simulink model "BACKSTEPPINGmasModosDeslisantes"  (R2025a)
settings: Solver=VariableStepAuto  StartTime=0.0  StopTime=10.0  RelTol=1e-3
InitFcn:
  | % --- INICIO DEL CÓDIGO InitFcn ---
  | 
  | % 1. (¡CAMBIA ESTO!) Asegúrate de que esta ruta sea correcta
  | addpath('C:/RoboDK/Matlab/');
  | 
  | % 2. Declarar las variables como globales para que Simulink las vea
  | global RDK;
  | global ROBOT;
  | 
  | % 3. Iniciar la conexión con RoboDK
  | RDK = Robolink();
  | 
  | % 4. (¡CAMBIA ESTO!) Pon el nombre exacto de tu robot en RoboDK
  | robot_name = 'Fanuc CRX-5iA';
  | ROBOT = RDK.Item(robot_name, RDK.ITEM_TYPE_ROBOT);
  | 
  | % 5. Comprobar que se encontró
  | if ~ROBOT.Valid()
  |     % Si el script falla aquí, es porque no encontró tu robot.
  |     error('No se encontró el robot: %s', robot_name);
  | end
  | 
  | % 6. Configurar el modo para simulación en tiempo real
  | RDK.setRunMode(RDK.RUNMODE_SIMULATE);
  | 
  | % 7. Mensaje de éxito
  | fprintf('¡RoboDK y el robot "%s" conectados a Simulink!\n', robot_name);
  | 
  | % --- FIN DEL CÓDIGO ---
libraries: robotmaniplib x1, robotsim3dlib x1, sim3dlib x1
settings Model: Creator=Sandro  LastModifiedBy=jaros

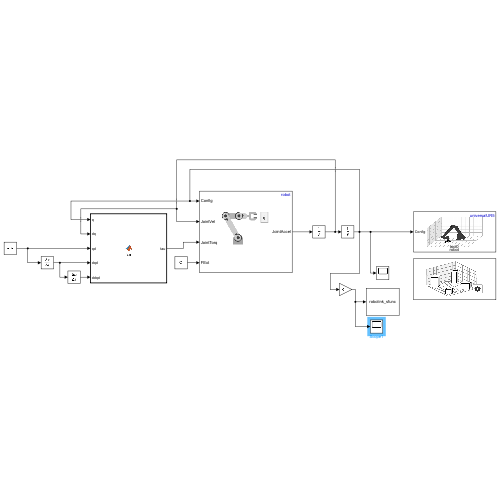
[thumbnail: Simulink's stored preview of the top-level diagram]
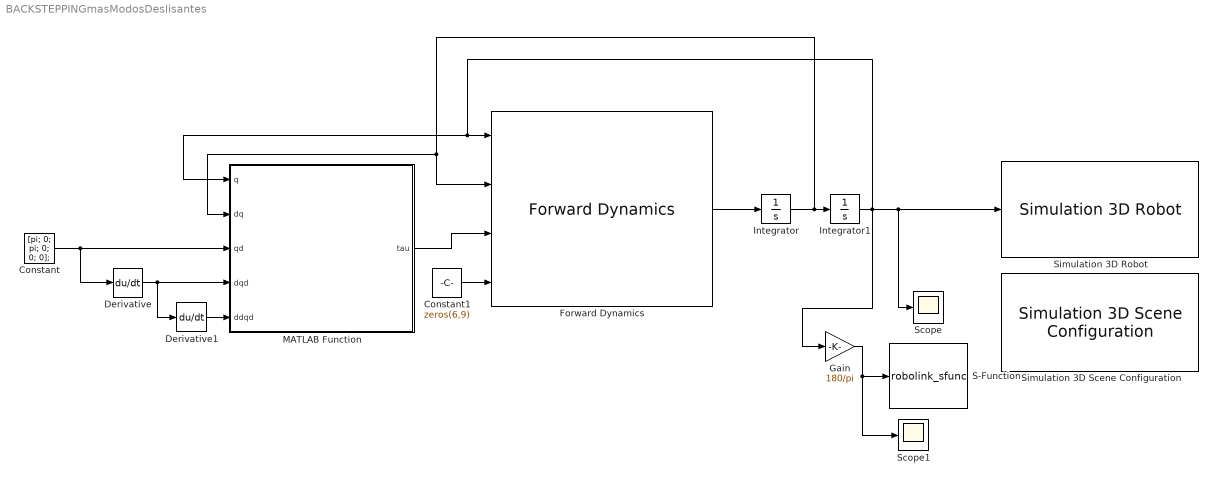
== system BACKSTEPPINGmasModosDeslisantes ==
  Constant : Constant  Value=[pi; 0; pi; 0; 0; 0];
  Constant1 : Constant  Value=zeros(6,9)
  Derivative : Derivative
  Derivative1 : Derivative
  Forward Dynamics : robotmaniplib/Forward Dynamics  RigidBodyTree=robot  SimulateUsing=Interpreted execution
  Gain : Gain  Gain=180/pi
  Integrator : Integrator
  Integrator1 : Integrator
  MATLAB Function : MATLAB Function  TreatAsAtomicUnit=on
  S-Function : S-Function  FunctionName=robolink_sfunc  SFunctionDeploymentMode=off  EnableBusSupport=off
  Scope : Scope
      settings: ActiveDisplayYMinimum=-0.47974053096022307  ActiveDisplayYMaximum=3.6061833571880464
  Scope1 : Scope
      settings: ActiveDisplayYMinimum=-27.538904576180038  ActiveDisplayYMaximum=207.08525853433974
  Simulation 3D Robot : robotsim3dlib/Simulation 3D Robot  actorInputType=Robot Library  RigidBodyTree=universalUR5  ActorName=robot  existActorChekBox=off  initialTrans=[0 0 0]  initialRot=[0 0 0]  initialConfig="[0  0  0  0  0  0]"  EndEffector=tool0  eeOffsetInpChekBox=off  eeTargetTrans=[0 0 0]  eeTargetRot=[0 0 0]  enableRegionGraspChekBox=off  regionGraspInpChekBox=off  eeTargTransDiff=[0.2 0.2 0.2]  eeTargRotDiff=[0 0 0]  enableVisualVisualization=on  enableCollisionVisualization=off  collisionGeomColor=[0 1 0]  collisionGeomTransp=0.1  inpConfEnbVal=on  inpGraspEnbVal=off  inpTransEnbVal=off  outConfEnbVal=off  outGraspEnbVal=off  outTransEnbVal=off  SampleTime=0.01  ActorType=SimulinkVehicle  ID=C  aMode=6  ActorTag=robot  Mesh=RigidBodyTree
  Simulation 3D Scene Configuration : sim3dlib/Simulation 3D Scene Configuration  Priority=0  ProjectFormat=Default Scenes  SceneDesc=Curved road  ProjectName=C:\Program Files\MATLAB\R2025a\toolbox\shared\sim3d_projects\automotive_project_windows\UE\WindowsNoEditor\VehicleSimulation.exe  ScenePath=/Game/Maps/EmptyScene  EnableOpenDRIVE=off  vehTagList={'<empty>';'Custom';'Scene Origin';'robot'}  vehTag=Scene Origin  AttachedCameraRelativeTranslation=[0 0 0]  FreeCameraDefaultInitialTranslation=[-6, 0, 2]  AttachedCameraRelativeRotation=[0 0 0]  FreeCameraDefaultInitialRotation=[0, -15, 0]  ViewpointName=Custom  FreeCameraInitialTranslation=[0 0 0]  ViewpointTranslation=[0 0 0]  FreeCameraInitialRotation=[0 0 0]  ViewpointRotation=[0 0 0]  OpVisEn=off  Ts=0.02  EnableWindow=on  EnableRemoteAccess=off  EnableWeather=off  SunAzimuth=90  SunAltitude=40.0  EnableGeospatialSun=off  Latitude=0  Longitude=0  Date=2023-01-01  Time=10:30:00  GeoTimeZone=-5.0  SunDaylightSaving=off  wind=1  clouds=10  EnableVolumetricClouds=off  CloudCoverage=0  CloudAltitude=6  fog=0  rain=0  RaindropsEffect=off  SnowDensity=0  EnableGeospatial=off  TilesetSource=Earth terrain  UseTrueOrigin=off  OriginHeight=200  OriginLatitude=40.744652  OriginLongitude=-73.988864  MapStyle=Aerial  AdditionalAssetIDs=[]  UseAdvancedSunSky=off  SolarTime=11  TimeZone=-5  Day=21  Month=9  Year=2022  UseDaylightSavingTime=on  DSTStartDay=10  DSTStartMonth=3  DSTEndDay=3  DSTEndMonth=11  DSTSwitchHour=2  sensorTag=MainCamera1  sensorId=1  sensorName=MainCamera1  mountLoc=Origin  offsetFlag=off  tmountOffset=[0, 0, 0]  rmountOffset=[0, 0, 0]  HorizontalResolution=1280  VerticalResolution=720  HorizontalFOV=60  mountPoint=[0 0 0]  mountOrientation=[0 0 0]  aMode=6  ID=1  GeoTrigger=Inactive  ViewNameList={'Custom'}  ViewTranslationList={'[0 0 0]'}  ViewRotationList={'[0 0 0]'}
      settings: LibrarySourceBlock=robotsim3dlib/Simulation 3D Scene Configuration
  wires:
  Forward Dynamics/1 -> Integrator/1
  Integrator/1 -> Forward Dynamics/2, MATLAB Function/2(dq), Integrator1/1
  Integrator1/1 -> Scope/1, Simulation 3D Robot/1, Gain/1, Forward Dynamics/1, MATLAB Function/1(q)
  Constant1/1 -> Forward Dynamics/4
  Constant/1 -> Derivative/1, MATLAB Function/3(qd)
  MATLAB Function/1(tau) -> Forward Dynamics/3
  Gain/1 -> Scope1/1, S-Function/1
  Derivative1/1 -> MATLAB Function/5(ddqd)
  Derivative/1 -> Derivative1/1, MATLAB Function/4(dqd)

== matlab function BACKSTEPPINGmasModosDeslisantes/MATLAB Function ==
  data: q input; dq input; qd input; tau output; dqd input; ddqd input
function tau = fcn(q, dq, qd, dqd, ddqd)
% ==========================================================
% Control Jerárquico Híbrido: Backstepping + Modos Deslizantes
% Diseñado para el robot Fanuc CRX-5iA
% ==========================================================
% Entradas:
%   q   -> posición actual [6x1] (rad)
%   dq  -> velocidad actual [6x1] (rad/s)
%   qd  -> posición deseada [6x1] (rad)
%   dqd -> velocidad deseada [6x1]
%   ddqd-> aceleración deseada [6x1]
%
% Salida:
%   tau -> torque de control [6x1]
% ==========================================================

% === Parámetros del control Backstepping ===
K1 = diag([40 40 30 20 15 10]);
K2 = diag([20 20 15 10 8 5]);

% === Cálculo de errores ===
e  = q - qd;          % error de posición
de = dq - dqd;        % error de velocidad

% === Ley Backstepping ===
tau_bs = -K1 * e - K2 * de;    % salida de la capa backstepping

% === Parámetros de la capa SMC ===
Lambda = diag([8 8 10 12 15 15]);
K = diag([15 10 8 5 4 3]);
phi = 0.1;  % zona muerta de saturación (reduce chattering)

% === Superficie deslizante ===
dq_r = dqd - Lambda*(q - qd);
s = dq - dq_r;

% Saturación para suavizar con phi
s_sat = zeros(6,1);
for i = 1:6
    if abs(s(i)) > phi
        s_sat(i) = sign(s(i));
    else
        s_sat(i) = s(i)/phi;
    end
end

% === Capa SMC ===
tau_smc = -K * s_sat;

% === Suma jerárquica de controladores ===
tau = tau_bs + tau_smc;

% === Limitador de torque ===
tau_max = [100 80 60 40 30 20]';
tau = clamp(tau, -tau_max, tau_max);

end


% ==========================================================
% ==== FUNCIONES AUXILIARES DENTRO DEL BLOQUE ==============
% ==========================================================
function y = clamp(x, min_val, max_val)
% Limita los valores de un vector entre rangos definidos
y = zeros(size(x));
for i = 1:length(x)
    if x(i) < min_val(i)
        y(i) = min_val(i);
    elseif x(i) > max_val(i)
        y(i) = max_val(i);
    else
        y(i) = x(i);
    end
end
end
